simulink library "ModifiedInductionMachine_lib"  (Simulink 8.1)
settings: Solver=ode45  StartTime=0.0  StopTime=10.0  RelTol=1e-3
undefined symbols (not defined in the file): gcbh, sps_rtmsupport
libraries: spsAsynchronousMachineModel x3
settings Model: Creator=ed12083  LastModifiedBy=ed12083

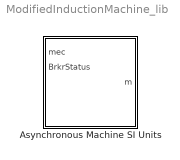
== system ModifiedInductionMachine_lib ==
  Asynchronous Machine SI Units : Subsystem  DialogController=POWERSYS.PowerSysDialog  LoadFcn=sps_rtmsupport('LoadFcn',gcbh);  StartFcn=sps_rtmsupport('StartFcn',gcbh);  StopFcn=sps_rtmsupport('StopFcn',gcbh);  mask(Asynchronous Machine){PresetModel=No, MechanicalLoad=Torque Tm, ShowDetailedParameters=on, RotorType=Squirrel-cage, ReferenceFrame=Stationary, NominalParameters=[ 136700/.92/.93, 480, 60 ], Stator=[ 0.029 0.226/377/1.5], Rotor=[ 0.022*3 0.226/377/1.5], Cage1=[ 0.022 0.226/377], Cage2=[ 0.022 0.226/377], Lm=13.04/377, Mechanical=[ 63.87 0  2 ], PolePairs=2, InitialConditions=[1 0 0 0 0 0 0 0], Units=SI, LoadFlowParameters=1492000, SimulateSaturation=off, Saturation=[14.03593122, 27.81365428, 53.79336849, 72.68890987, 97.98006896, 148.6815601, 215.7428561, 302.9841135, 420.4778367 ; 230, 322, 414, 460, 506, 552, 598, 644, 690], TsPowergui=0, TsBlock=-1, IterativeModel=Trapezoidal non iterative, Pmec=0}
      mask prompts: PresetModel "Preset model:"; MechanicalLoad "Mechanical input:"; ShowDetailedParameters "Show detailed parameters"; RotorType "Rotor type:"; ReferenceFrame "Reference frame:"; NominalParameters "Nominal power, voltage (line-line), and frequency [ Pn(VA),Vn(Vrms),fn(Hz) ]:"; Stator "Stator resistance and inductance[ Rs(ohm)  Lls(H) ]:"; Rotor "Rotor resistance and inductance [ Rr'(ohm)  Llr'(H) ]:"; Cage1 "Cage 1 resistance and inductance  [ Rr1' (ohm)  Llr1' (H) ]:"; Cage2 "Cage 2 resistance and inductance  [ Rr2' (ohm)  Llr2' (H) ]:"; Lm "Mutual inductance Lm (H):"; Mechanical "Inertia, friction factor, pole pairs [ J(kg.m^2)  F(N.m.s)   p() ]:"; PolePairs "Pole pairs p ():"; InitialConditions "Initial conditions"; Units "Mask units:"; LoadFlowParameters "Load flow Parameters"; SimulateSaturation "Simulate saturation"; Saturation "Saturation Parameters [i1,i2,... (Arms) ; v1,v2,...(VrmsLL)]"; TsPowergui "Sample time of powergui block"; TsBlock "Sample time (-1 for inherited)"; IterativeModel "Discrete solver model"; Pmec "Mechanical power (W)"
      mask help: Implements a three-phase asynchronous machine (wound rotor, squirrel cage or double squirrel cage) modeled in a selectable dq reference frame (rotor, stator, or synchronous). Stator and rotor windings are connected in wye to an internal neutral point.
      mask init:
      | block = gcb;
      | [Ts,SM,WantBlockChoice,X,Y,txt] = powericon('AsynchronousMachineInit',block,TsPowergui,TsBlock,MechanicalLoad,RotorType,ReferenceFrame,NominalParameters,Stator,Rotor,Cage1,Cage2,Lm,Mechanical,PolePairs,InitialConditions,Units,SimulateSaturation,Saturation,IterativeModel);
      | powericon('SetInternalModels','set',block,WantBlockChoice); sps_rtmsupport('parametereditingmodes',block, [1 2 3 4 5 15 17 21]); 
      | powericon('ShaftInput',(block));
      settings: AttributesFormatString=\n  CopyFcn=sps_rtmsupport('CopyFcn',gcbh); powericon('psbloadfunction',gcbh,'gotofrom','UpdateGotoTag');  DeleteFcn=sps_rtmsupport('DeleteFcn',gcbh);  UndoDeleteFcn=sps_rtmsupport('UndoDeleteFcn',gcbh);  ModelCloseFcn=sps_rtmsupport('ModelCloseFcn',gcbh);  PreSaveFcn=sps_rtmsupport('PreSaveFcn',gcbh);  PostSaveFcn=sps_rtmsupport('PostSaveFcn',gcbh);  NameChangeFcn=sps_rtmsupport('NameChangeFcn',gcbh);  PreCopyFcn=sps_rtmsupport('PreCopyFcn',gcbh);  OpenFcn=sps_rtmsupport('OpenFcn',gcbh, [1 2 3 4 5 15 17 21]);  CloseFcn=sps_rtmsupport('CloseFcn',gcbh);  PreDeleteFcn=sps_rtmsupport('PreDeleteFcn',gcbh);
      mask Help: helpview(psbhelp);
      mask TypeOptions PresetModel: No | 01:  5 HP   460 V 60Hz 1750 RPM            | 02:  10 HP  460 V 60Hz 1760 RPM           | 03:  20 HP  460 V 60Hz 1760 RPM           | 04:  50 HP  460 V 60Hz 1780 RPM           | 05:  100 HP 460 V 60Hz 1780 RPM          | 06:  150 HP 460 V 60Hz 1785 RPM          | 07:  200 HP 460 V 60Hz 1785 RPM          | 08:  5 HP   575 V 60Hz 1750 RPM            | 09:  10 HP  575 V 60Hz 1760 RPM           | 10:  20 HP  575 V 60Hz 1765 RPM           | 11:  50 HP  575 V 60Hz 1775 RPM           | 12:  100 HP 575 V 60Hz 1780 RPM          | 13:  150 HP 575 V 60Hz 1785 RPM          | 14:  200 HP 575 V 60Hz 1785 RPM          | 15:  5.4 HP (4KW)   400 V  50Hz 1430 RPM   | 16:  10 HP (7.5KW)  400 V 50Hz 1440 RPM  | 17:  20 HP (15KW)   400 V 50Hz 1460 RPM   | 18:  50 HP (37KW)   400 V 50Hz 1480 RPM   | 19:  100 HP (75KW)  400 V 50Hz 1484 RPM  | 20:  150 HP (110KW) 400 V 50Hz 1487 RPM | 21:  215 HP (160KW) 400 V 50Hz 1487 RPM
      mask Callback PresetModel: powericon('AsynchronousMachineCback',gcb,'SI');
      mask TypeOptions MechanicalLoad: Torque Tm | Speed w | Mechanical rotational port
      mask Callback MechanicalLoad: %powericon('AsynchronousMachineCback',gcb);
      mask Callback ShowDetailedParameters: %powericon('AsynchronousMachineCback',gcb);
      mask TypeOptions RotorType: Wound | Squirrel-cage | Double squirrel-cage
      mask Callback RotorType: powericon('AsynchronousMachineCback',gcb,'SI','RotorType');
      mask TypeOptions ReferenceFrame: Rotor | Stationary | Synchronous
      mask TypeOptions Units: SI
      mask Callback SimulateSaturation: powericon('AsynchronousMachineCback',gcb,'SI');
      mask TypeOptions IterativeModel: Trapezoidal non iterative | Trapezoidal iterative (alg. loop) | Forward Euler
      mask Callback Pmec: sps_rtmsupport('parametereditingmodes',gcbh, [1 2 3 4 5 15 17 21]);
      mask Display:
      | plot(X.p1,Y.p1,X.p2,Y.p2,X.p3,Y.p3,X.p4,Y.p4,X.p5,Y.p5,X.p6,Y.p6,X.p7,Y.p7,X.p8,Y.p8,X.p9,Y.p9,X.p10,Y.p10)
      | color('blue');
      | plot(X.p11,Y.p11);
      | plot(X.p12,Y.p12);
      | if strcmp(get_param(block,'MechanicalLoad'),'Mechanical rotational port');
      | else
      |     port_label('input',1,SM.PortLabel)
      | end
      | text(0,20,txt,'HorizontalAlignment','Center')

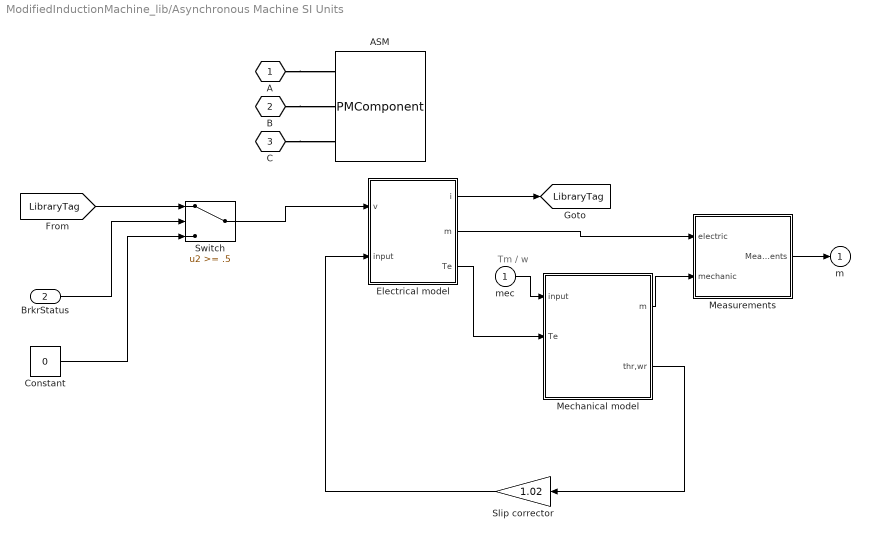
== system ModifiedInductionMachine_lib/Asynchronous Machine SI Units ==
  note: Tm / w
  mec : Inport
  BrkrStatus : Inport  Port=2
  ASM : PMComponent  PhysicalDomain=powersysdomain  LeftPortType=p1  RightPortType=p1  LConnTagsString=A|B|C  RConnTagsString=a|b|c  mask(InnerPowersysBlock){}
  Constant : Constant  Value=0
  Electrical model : Subsystem  BlockChoice=Continuous
      settings: AttributesFormatString=%<BlockChoice>  TemplateBlock=spsAsynchronousMachineModel/Electrical model  MemberBlocks=Continuous,Continuous double-cage,Discrete,Discrete Trapezoidal,Discrete double-cage,Phasor,Phasor double-cage
  Measurements : Subsystem  BlockChoice=Single-cage SI
      settings: AttributesFormatString=%<BlockChoice>  TemplateBlock=spsAsynchronousMachineModel/Measurements  MemberBlocks=Double-cage SI,Double-cage pu,Single-cage SI,Single-cage pu
  Mechanical model : Subsystem  BlockChoice=Continuous Tm input
      settings: AttributesFormatString=%<BlockChoice>  TemplateBlock=spsAsynchronousMachineModel/Mechanical model  MemberBlocks=Continuous Tm input,Continuous w input,Discrete Tm input,Discrete Tm input Trapezoidal,Discrete w input,Phasor Shaft input,Phasor Tm input,Phasor w input,Shaft input,Shaft input BAL
  Slip corrector : Gain  Gain=1.02
  Switch : Switch  Threshold=.5
  A : PMIOPort  Port=1  Side=Left
  B : PMIOPort  Port=2  Side=Left
  C : PMIOPort  Port=3  Side=Left
  m : Outport  InitialOutput=0
  tag scope: LibraryTag=global
  wires:
  BrkrStatus/1 -> Switch/2
  Constant/1 -> Switch/3
  Switch/1 -> Electrical model/1(v)
  [LibraryTag] -> Switch/1
  Mechanical model/2(thr,wr) -> Slip corrector/1
  Mechanical model/1(m) -> Measurements/2(mechanic)
  Electrical model/2(m) -> Measurements/1(electric)
  Electrical model/1(i) -> [LibraryTag]
  Measurements/1(Measurements) -> m/1
  Electrical model/3(Te) -> Mechanical model/2(Te)
  mec/1 -> Mechanical model/1(input)
  Slip corrector/1 -> Electrical model/2(input)
  connections:
  C/RConn1 -- ASM/LConn3
  B/RConn1 -- ASM/LConn2
  A/RConn1 -- ASM/LConn1

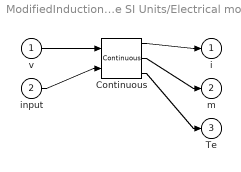
== system ModifiedInductionMachine_lib/Asynchronous Machine SI Units/Electrical model ==
  v : Inport
  input : Inport  Port=2
  Continuous : spsAsynchronousMachineModel/Continuous
  i : Outport
  m : Outport  Port=2
  Te : Outport  Port=3
  wires:
  v/1 -> Continuous/1
  input/1 -> Continuous/2
  Continuous/1 -> i/1
  Continuous/2 -> m/1
  Continuous/3 -> Te/1

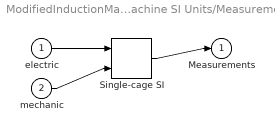
== system ModifiedInductionMachine_lib/Asynchronous Machine SI Units/Measurements ==
  electric : Inport
  mechanic : Inport  Port=2
  Single-cage SI : spsAsynchronousMachineModel/Single-cage SI
  Measurements : Outport
  wires:
  Single-cage SI/1 -> Measurements/1
  mechanic/1 -> Single-cage SI/2
  electric/1 -> Single-cage SI/1

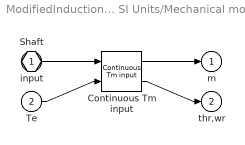
== system ModifiedInductionMachine_lib/Asynchronous Machine SI Units/Mechanical model ==
  input : Inport
  Te : Inport  Port=2
  Continuous Tm input : spsAsynchronousMachineModel/Continuous Tm input
  Shaft : PMIOPort  Port=1  Side=Left
  m : Outport
  thr,wr : Outport  Port=2
  wires:
  input/1 -> Continuous Tm input/1
  Te/1 -> Continuous Tm input/2
  Continuous Tm input/1 -> m/1
  Continuous Tm input/2 -> thr,wr/1
